simulink model "LinearVCCS"  (R2024b)
settings: Solver=VariableStepAuto  StartTime=0.0  StopTime=10.0  RelTol=1e-3
libraries: fl_lib x2
settings Model: Creator=JesseJabezArendse  LastModifiedBy=JesseJabezArendse

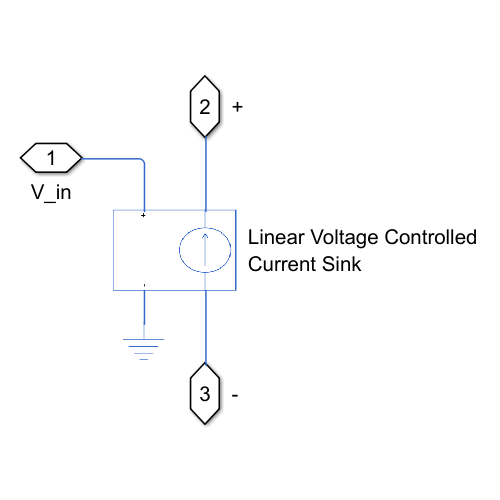
[thumbnail: Simulink's stored preview of the top-level diagram]
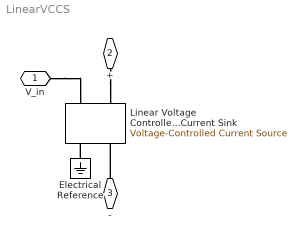
== system LinearVCCS ==
  Electrical Reference : fl_lib/Electrical/Electrical Elements/Electrical Reference
  Linear Voltage Controlled Current Sink : fl_lib/Electrical/Electrical Sources/Voltage-Controlled Current Source  K=0.1/3.3 1/Ohm  v1_specify=off  v1_priority=None  v1=0 V  v1_nominal_specify=off  v1_nominal_value=1  v1_nominal_unit=V  i2_specify=off  i2_priority=None  i2=0 A  i2_nominal_specify=off  i2_nominal_value=1  i2_nominal_unit=A
      settings: InternalSimscapePortConfiguration="{\"Bottom\":[],\"Left\":[{\"id\":\"p1\",\"label\":\"+\",\"type\":\"foundation.electrical.electrical\"},{\"id\":\"head\",\"label\":\"\",\"type\":\"foundation.electrical.electrical\"}],\"Right\":[{\"id\":\"n1\",\"label\":\"-\",\"type\":\"foundation.electrical.electrical\"},{\"id\":\"tail\",\"label\":\"\",\"type\":\"foundation.electrical.electrical\"}],\"Top\":[]}"
  V_in : PMIOPort  Side=Left
  + : PMIOPort  Port=2  Side=Left
  - : PMIOPort  Port=3  Side=Left
  connections:
  V_in/RConn1 -- Linear Voltage Controlled Current Sink/LConn1
  Electrical Reference/LConn1 -- Linear Voltage Controlled Current Sink/RConn1
  +/RConn1 -- Linear Voltage Controlled Current Sink/LConn2
  -/RConn1 -- Linear Voltage Controlled Current Sink/RConn2
